simulink model "MotorCD1v1"  (Simulink 5.0)
settings: Solver=ode45  StartTime=0.0  StopTime=40  RelTol=1e-3
values from neighbouring files (symbols this model uses):
  B = 20    [MasaEjemplo1_valores.m]    (also in VariablesMotorCD.m = 0.01)
  J = 0.02    [VariablesMotorCD.m]
  Kb = 0.11    [VariablesMotorCD.m]
  Ki = 0.11    [VariablesMotorCD.m]
  La = 0.02    [VariablesMotorCD.m]
  Ra = 2    [VariablesMotorCD.m]
settings Model: LastModifiedBy=gaby

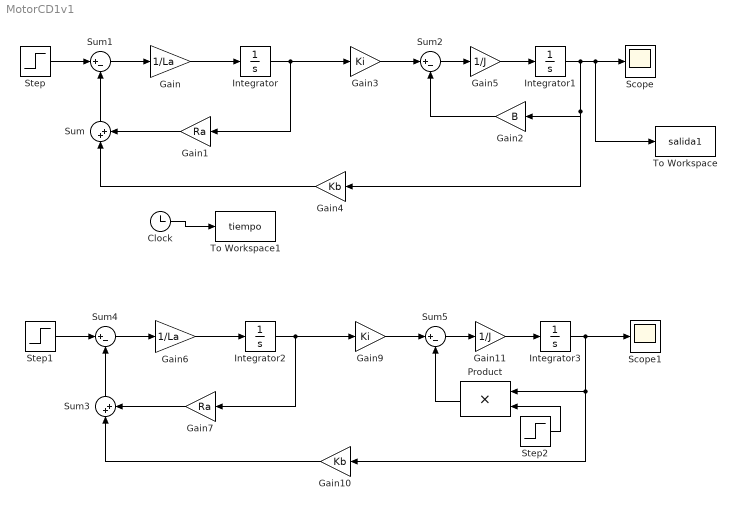
== system MotorCD1v1 ==
  Clock : Clock
      settings: Decimation=10
  Gain : Gain  Gain=1/La  SaturateOnIntegerOverflow=on
  Gain1 : Gain  Orientation=left  Gain=Ra  SaturateOnIntegerOverflow=on
  Gain10 : Gain  Orientation=left  Gain=Kb  SaturateOnIntegerOverflow=on
  Gain11 : Gain  Gain=1/J  SaturateOnIntegerOverflow=on
  Gain2 : Gain  Orientation=left  Gain=B  SaturateOnIntegerOverflow=on
  Gain3 : Gain  Gain=Ki  SaturateOnIntegerOverflow=on
  Gain4 : Gain  Orientation=left  Gain=Kb  SaturateOnIntegerOverflow=on
  Gain5 : Gain  Gain=1/J  SaturateOnIntegerOverflow=on
  Gain6 : Gain  Gain=1/La  SaturateOnIntegerOverflow=on
  Gain7 : Gain  Orientation=left  Gain=Ra  SaturateOnIntegerOverflow=on
  Gain9 : Gain  Gain=Ki  SaturateOnIntegerOverflow=on
  Integrator{,1..3} (4 alike) : Integrator
  Product : Product  Orientation=left  SaturateOnIntegerOverflow=on
  Scope : Scope
  Scope1 : Scope
  Step : Step  Time=0  After=20  SampleTime=0
  Step1 : Step  Time=0  After=20  SampleTime=0
  Step2 : Step  Time=1500*0.01*0.02/(0.11)^2  Before=0.01  After=0.5*0.01  SampleTime=0
  Sum : Sum  Orientation=up  Inputs=|++  SaturateOnIntegerOverflow=on
  Sum{1..2,4..5} (4 alike) : Sum  Inputs=|+-  SaturateOnIntegerOverflow=on
  Sum3 : Sum  Orientation=up  Inputs=|++  SaturateOnIntegerOverflow=on
  To Workspace : ToWorkspace  VariableName=salida1  SampleTime=-1  SaveFormat=Array
  To Workspace1 : ToWorkspace  VariableName=tiempo  SampleTime=-1  SaveFormat=Array
  wires:
  Sum1/1 -> Gain/1
  Gain/1 -> Integrator/1
  Integrator/1 -> Gain3/1, Gain1/1
  Gain3/1 -> Sum2/1
  Sum2/1 -> Gain5/1
  Gain5/1 -> Integrator1/1
  Gain1/1 -> Sum/2
  Sum/1 -> Sum1/2
  Gain2/1 -> Sum2/2
  Integrator1/1 -> Gain4/1, Gain2/1, Scope/1, To Workspace/1
  Gain4/1 -> Sum/1
  Step/1 -> Sum1/1
  Sum4/1 -> Gain6/1
  Gain6/1 -> Integrator2/1
  Integrator2/1 -> Gain9/1, Gain7/1
  Gain9/1 -> Sum5/1
  Sum5/1 -> Gain11/1
  Gain11/1 -> Integrator3/1
  Gain7/1 -> Sum3/2
  Sum3/1 -> Sum4/2
  Integrator3/1 -> Scope1/1, Gain10/1, Product/1
  Gain10/1 -> Sum3/1
  Step1/1 -> Sum4/1
  Product/1 -> Sum5/2
  Step2/1 -> Product/2
  Clock/1 -> To Workspace1/1
